simulink library "thc"  (R2021b)
settings: Solver=VariableStepAuto  StartTime=0.0  StopTime=10.0  RelTol=1e-3
undefined symbols (not defined in the file): ATHC_APTCQA_X_C, ATHC_APTCQB_X_C, ATHC_dAy_X_C, ATHC_Qeq_X_kmh, ATHC_VbaseC_X_C, ATHC_VbaseC_Y_W, ATHC_VbaseD_X_C, ATHC_VbaseH_X_C, FALSE, KTHC_ACMaxMinT_sec, KTHC_aDeice_K, KTHC_AGSDefLv_K, KTHC_AGSLv1_K, KTHC_AGSLv2_K, KTHC_AGSLv3_K, KTHC_AGSLv4_K, KTHC_AGSLv5_K, KTHC_AirIntUpdateT_sec, KTHC_APTCOneZoneMax_W, KTHC_APTCPeriod_cnt, KTHC_APTCPWMEN_flg, KTHC_APTCQMaxC_W, KTHC_APTCQminC_W, KTHC_APTCQminD_W, KTHC_APTCQminRe1_W, KTHC_APTCQminRe_W, KTHC_APTCQoffT_cnt, KTHC_APTCQonT_cnt, KTHC_APTCRiLeMaxDff_W, KTHC_APTCRiLeMinDff_W, KTHC_BatCoolT_cnt, KTHC_BatInTempDef_C, KTHC_bDeice_K, KTHC_CompMaxDeice_rpm, KTHC_CompMinDeice_rpm, KTHC_CompSotxvOp_K, KTHC_CompSotxvOpLow_rpm, KTHC_CompSpdmax_rpm, KTHC_CompSpdmaxBC1_rpm, KTHC_CompSpdmaxBC_rpm, KTHC_CompSpdmid1_rpm, KTHC_CompSpdmid2_rpm, KTHC_CompSpdmid3_rpm, KTHC_CompSpdmid_rpm, KTHC_CompSpdmin_rpm, KTHC_DAPTCQ1_W, KTHC_DAPTCQ2_W, KTHC_DAPTCQ3_W, KTHC_DcChSetTemp_C, KTHC_DehumidityEN_flg, KTHC_DeiceCycTime_K, KTHC_DriveLevelWPTCBAH1_W, KTHC_DriveLevelWPTCBAH2_W, KTHC_DriveLevelWPTCBAH3_W, KTHC_DriveLevelWPTCBAH4_W, KTHC_DriverSeatPos_flg, KTHC_DriveT1MinBAH_C, KTHC_DriveT2MaxBAH_C, KTHC_DriveT2MinBAH_C, KTHC_DriveT3MaxBAH_C ... (+379)
libraries: simulink x489
(part 14 of 17)

== system thc/THC/ThermalControl/THCM_Conctrl/CompCtrl/Enabled Subsystem ==
  sigSetTempZon1StC : Inport
  Tincar : Inport  Port=2
  Tamb : Inport  Port=3
  VINP_SmartEcoModeSW_flg : Inport  Port=4
  Enable : EnablePort
  Chart : Stateflow chart  TreatAsAtomicUnit=on
  Constant : Constant  Value=KTHC_DTymin1_K
  Constant1 : Constant  Value=KTHC_Tambmin_C
  Constant10 : Constant  Value=KTHC_T4Maxamb_C
  Constant11 : Constant  Value=KTHC_T2Minamb_C
  Constant12 : Constant  Value=KTHC_T3Minamb_C
  Constant13 : Constant  Value=KTHC_T4Minamb_C
  Constant14 : Constant  Value=KTHC_T5Minamb_C
  Constant3 : Constant  Value=KTHC_DTymin2_K
  Constant4 : Constant  Value=KTHC_DTymin3_K
  Constant5 : Constant  Value=KTHC_DTymin4_K
  Constant6 : Constant  Value=KTHC_DTymin5_K
  Constant7 : Constant  Value=KTHC_T1Maxamb_C
  Constant8 : Constant  Value=KTHC_T2Maxamb_C
  Constant9 : Constant  Value=KTHC_T3Maxamb_C
  Product : Product
  Relational Operator1 : RelationalOperator  OutDataTypeStr=boolean  RndMeth=Simplest
  Sum : Sum  Inputs=|+-
  Switch : Switch  Criteria=u2 > Threshold
  Switch1 : Switch  Criteria=u2 > Threshold
  TincarCe : Outport
  TincarCset : Outport  Port=2
  wires:
  sigSetTempZon1StC/1 -> Sum/1, TincarCset/1  "sigSetTempZon1StC"
  Tincar/1 -> Sum/2
  Switch1/1 -> Switch/1
  Switch/1 -> TincarCe/1
  Sum/1 -> Switch/3, Product/2, Switch1/3
  Constant1/1 -> Relational Operator1/2
  Relational Operator1/1 -> Switch/2
  Tamb/1 -> [Tamb]
  [Tamb] -> Chart/1(Tamb)
  Constant/1 -> Chart/2(KTHC_DTymin1_K)
  Constant3/1 -> Chart/3(KTHC_DTymin2_K)
  Constant4/1 -> Chart/4(KTHC_DTymin3_K)
  Constant5/1 -> Chart/5(KTHC_DTymin4_K)
  Constant6/1 -> Chart/6(KTHC_DTymin5_K)
  Constant7/1 -> Chart/7(KTHC_T1Maxamb_C)
  Constant8/1 -> Chart/8(KTHC_T2Maxamb_C)
  Constant9/1 -> Chart/9(KTHC_T3Maxamb_C)
  Constant10/1 -> Chart/10(KTHC_T4Maxamb_C)
  Constant11/1 -> Chart/11(KTHC_T2Minamb_C)
  Constant12/1 -> Chart/12(KTHC_T3Minamb_C)
  Constant13/1 -> Chart/13(KTHC_T4Minamb_C)
  Constant14/1 -> Chart/14(KTHC_T5Minamb_C)
  Chart/1(DTymin) -> [DTymin]
  [DTymin] -> Product/1
  [Tamb] -> Relational Operator1/1
  Product/1 -> Switch1/1
  VINP_SmartEcoModeSW_flg/1 -> Switch1/2

== system thc/THC/ThermalControl/THCM_Conctrl/CompCtrl/Enabled Subsystem1 ==
  TBMax : Inport
  Bat_In_Temp : Inport  Port=2
  Enable : EnablePort
  Chart : Stateflow chart  TreatAsAtomicUnit=on
  Constant : Constant  Value=KTHC_T1MaxBC_C
  Constant1 : Constant  Value=KTHC_T1winSetpointBC_C
  Constant10 : Constant  Value=KTHC_T3MinBC_C
  Constant11 : Constant  Value=KTHC_T3MaxBC_C
  Constant12 : Constant  Value=KTHC_T4MinBC_C
  Constant14 : Constant  Value=KTHC_T4MaxBC_C
  Constant15 : Constant  Value=KTHC_T5MinBC_C
  Constant2 : Constant  Value=KTHC_T2winSetpointBC_C
  Constant3 : Constant  Value=KTHC_T3winSetpointBC_C
  Constant4 : Constant  Value=KTHC_T4winSetpointBC_C
  Constant5 : Constant  Value=KTHC_T5winSetpointBC_C
  Constant8 : Constant  Value=KTHC_T2MinBC_C
  Constant9 : Constant  Value=KTHC_T2MaxBC_C
  Sum : Sum  Inputs=|+-
  BatIne : Outport
  BatInset : Outport  Port=2
  wires:
  TBMax/1 -> Chart/1(TBMax)
  Chart/1(Bat_In_TempSetPoint) -> BatInset/1, Sum/1  "Bat_In_TempSetPoint"
  Bat_In_Temp/1 -> Sum/2
  Sum/1 -> BatIne/1
  Constant/1 -> Chart/2(KTHC_T1MaxBC_C)
  Constant8/1 -> Chart/3(KTHC_T2MinBC_C)
  Constant9/1 -> Chart/4(KTHC_T2MaxBC_C)
  Constant10/1 -> Chart/5(KTHC_T3MinBC_C)
  Constant11/1 -> Chart/6(KTHC_T3MaxBC_C)
  Constant12/1 -> Chart/7(KTHC_T4MinBC_C)
  Constant14/1 -> Chart/8(KTHC_T4MaxBC_C)
  Constant15/1 -> Chart/9(KTHC_T5MinBC_C)
  Constant1/1 -> Chart/10(KTHC_T1winSetpointBC_C)
  Constant2/1 -> Chart/11(KTHC_T2winSetpointBC_C)
  Constant3/1 -> Chart/12(KTHC_T3winSetpointBC_C)
  Constant4/1 -> Chart/13(KTHC_T4winSetpointBC_C)
  Constant5/1 -> Chart/14(KTHC_T5winSetpointBC_C)

== system thc/THC/ThermalControl/THCM_Conctrl/CompCtrl/Enabled Subsystem2 ==
  sigSetTempZon1St : Inport
  Tincar : Inport  Port=2
  Enable : EnablePort
  Sum : Sum  Inputs=|+-
  Tincare : Outport
  Tincarset : Outport  Port=2
  wires:
  sigSetTempZon1St/1 -> Tincarset/1, Sum/1
  Sum/1 -> Tincare/1
  Tincar/1 -> Sum/2

== system thc/THC/ThermalControl/THCM_Conctrl/CompCtrl/Enabled Subsystem3 ==
  PT_Low_P2 : Inport
  PT_ Low_P2Setpoint : Inport  Port=2
  Enable : EnablePort
  Sum : Sum  Inputs=|+-
  PTLowP2e : Outport
  wires:
  PT_Low_P2/1 -> Sum/2
  PT_ Low_P2Setpoint/1 -> Sum/1
  Sum/1 -> PTLowP2e/1

== system thc/THC/ThermalControl/THCM_Conctrl/CompCtrl/Enabled Subsystem4 ==
  PT_High_P : Inport
  PT_High_PSetpoint : Inport  Port=2
  Enable : EnablePort
  Sum : Sum  Inputs=|+-
  PT_High_Pe : Outport
  wires:
  Sum/1 -> PT_High_Pe/1
  PT_High_PSetpoint/1 -> Sum/1
  PT_High_P/1 -> Sum/2

== system thc/THC/ThermalControl/THCM_Conctrl/CompCtrl/Enabled Subsystem5 ==
  PT_Low_P1 : Inport
  PT_Low_P1Setpoint : Inport  Port=2
  Enable : EnablePort
  Sum : Sum  Inputs=|+-
  PT_Low_Pe : Outport
  wires:
  PT_Low_P1/1 -> Sum/2
  PT_Low_P1Setpoint/1 -> Sum/1
  Sum/1 -> PT_Low_Pe/1

== system thc/THC/ThermalControl/THCM_Conctrl/EXV1Ctrl/EXV1PIControl ==
  x : Inport
  Reset : Inport  Port=2
  VTHC_KpEXV1SH_K : Inport  Port=3
  VTHC_KiEXV1SH_K : Inport  Port=4
  Add : Sum
  Add1 : Sum
  Constant : Constant  Value=0
  Product : Product
  Product1 : Product
  Saturation : Saturate  UpperLimit=0.1  LowerLimit=-0.9
  Switch : Switch  Criteria=u2 > Threshold
  Ts : Gain  Gain=0.1
  Unit Delay1 : UnitDelay  SampleTime=-1  HasFrameUpgradeWarning=on
  VTHC_EXV1P_K : Outport
  VTHC_EXV1I_K : Outport  Port=2
  VTHC_EXV1U_K : Outport  Port=3
  wires:
  Constant/1 -> Switch/1
  x/1 -> Product/2, Product1/1
  Product/1 -> VTHC_EXV1P_K/1, Add/1  "VTHC_EXV1P_K"
  Add/1 -> VTHC_EXV1U_K/1
  Add1/1 -> Unit Delay1/1
  Product1/1 -> Ts/1
  Switch/1 -> VTHC_EXV1I_K/1, Add/2, Add1/2  "VTHC_EXV1I_K"
  Unit Delay1/1 -> Saturation/1
  VTHC_KpEXV1SH_K/1 -> Product/1
  VTHC_KiEXV1SH_K/1 -> Product1/2
  Reset/1 -> Switch/2
  Saturation/1 -> Switch/3
  Ts/1 -> Add1/1  "VTHC_EXV1I_K"

== system thc/THC/ThermalControl/THCM_Conctrl/EXV2Ctrl/EXV2PIControl ==
  x : Inport
  Reset : Inport  Port=2
  VTHC_KpEXV2_K : Inport  Port=3
  VTHC_KiEXV2_K : Inport  Port=4
  Add : Sum
  Add1 : Sum
  Constant : Constant  Value=0
  Equal : RelationalOperator  Operator=~=  OutDataTypeStr=boolean  RndMeth=Simplest
  Product : Product
  Product1 : Product
  Saturation : Saturate  UpperLimit=0.1  LowerLimit=-0.9
  Switch : Switch  Criteria=u2 > Threshold
  Ts : Gain  Gain=0.1
  Unit Delay : UnitDelay  SampleTime=-1  HasFrameUpgradeWarning=on
  Unit Delay1 : UnitDelay  SampleTime=-1  HasFrameUpgradeWarning=on
  VTHC_EXV2P_K : Outport
  VTHC_EXV2I_K : Outport  Port=2
  VTHC_EXV2U_K : Outport  Port=3
  wires:
  Unit Delay/1 -> Equal/2
  Equal/1 -> Switch/2
  Constant/1 -> Switch/1
  x/1 -> Product1/1, Product/2
  Product/1 -> VTHC_EXV2P_K/1, Add/1  "VTHC_EXV2P_K"
  Add/1 -> VTHC_EXV2U_K/1
  Add1/1 -> Unit Delay1/1
  Product1/1 -> Ts/1
  Switch/1 -> VTHC_EXV2I_K/1, Add/2, Add1/2  "VTHC_EXV2I_K"
  Reset/1 -> Unit Delay/1, Equal/1
  VTHC_KpEXV2_K/1 -> Product/1
  VTHC_KiEXV2_K/1 -> Product1/2
  Ts/1 -> Add1/1
  Unit Delay1/1 -> Saturation/1
  Saturation/1 -> Switch/3

== system thc/THC/ThermalControl/THCM_Conctrl/Subsystem1/SensorErrorHandle1 ==
  DataIn : Inport
  SensorError : Inport  Port=2
  PresetValue : Inport  Port=3
  Constant : Constant  Value=KTHC_ErrHandleEN_flg
  Logical Operator : Logic  AllPortsSameDT=off  OutDataTypeStr=boolean
  Switch : Switch  Criteria=u2 > Threshold
  DataOut : Outport
  wires:
  PresetValue/1 -> Switch/1
  DataIn/1 -> Switch/3
  Switch/1 -> DataOut/1
  Logical Operator/1 -> Switch/2
  SensorError/1 -> Logical Operator/1
  Constant/1 -> Logical Operator/2

== system thc/THC/ThermalControl/THCM_Conctrl/Subsystem1/SensorErrorHandle2 ==
  DataIn : Inport
  SensorError : Inport  Port=2
  PresetValue : Inport  Port=3
  Constant : Constant  Value=KTHC_ErrHandleEN_flg
  Logical Operator : Logic  AllPortsSameDT=off  OutDataTypeStr=boolean
  Switch : Switch  Criteria=u2 > Threshold
  DataOut : Outport
  wires:
  Constant/1 -> Logical Operator/2
  SensorError/1 -> Logical Operator/1
  Logical Operator/1 -> Switch/2
  Switch/1 -> DataOut/1
  DataIn/1 -> Switch/3
  PresetValue/1 -> Switch/1

== system thc/THC/ThermalControl/THCM_Conctrl/Subsystem1/SensorErrorHandle3 ==
  DataIn : Inport
  SensorError : Inport  Port=2
  PresetValue : Inport  Port=3
  Constant : Constant  Value=KTHC_ErrHandleEN_flg
  Logical Operator : Logic  AllPortsSameDT=off  OutDataTypeStr=boolean
  Switch : Switch  Criteria=u2 > Threshold
  DataOut : Outport
  wires:
  PresetValue/1 -> Switch/1
  DataIn/1 -> Switch/3
  Switch/1 -> DataOut/1
  Logical Operator/1 -> Switch/2
  SensorError/1 -> Logical Operator/1
  Constant/1 -> Logical Operator/2

== system thc/THC/ThermalControl/THCM_Conctrl/Subsystem1/SensorErrorHandle4 ==
  DataIn : Inport
  SensorError : Inport  Port=2
  PresetValue : Inport  Port=3
  Constant : Constant  Value=KTHC_ErrHandleEN_flg
  Logical Operator : Logic  AllPortsSameDT=off  OutDataTypeStr=boolean
  Switch : Switch  Criteria=u2 > Threshold
  DataOut : Outport
  wires:
  Constant/1 -> Logical Operator/2
  SensorError/1 -> Logical Operator/1
  Logical Operator/1 -> Switch/2
  Switch/1 -> DataOut/1
  DataIn/1 -> Switch/3
  PresetValue/1 -> Switch/1

== system thc/THC/ThermalControl/THCM_Conctrl/Subsystem1/SensorErrorHandle5 ==
  DataIn : Inport
  SensorError : Inport  Port=2
  PresetValue : Inport  Port=3
  Constant : Constant  Value=KTHC_ErrHandleEN_flg
  Logical Operator : Logic  AllPortsSameDT=off  OutDataTypeStr=boolean
  Switch : Switch  Criteria=u2 > Threshold
  DataOut : Outport
  wires:
  PresetValue/1 -> Switch/1
  DataIn/1 -> Switch/3
  Switch/1 -> DataOut/1
  Logical Operator/1 -> Switch/2
  SensorError/1 -> Logical Operator/1
  Constant/1 -> Logical Operator/2

== system thc/THC/ThermalControl/THCM_Conctrl/Subsystem1/SensorErrorHandle9 ==
  DataIn : Inport
  SensorError : Inport  Port=2
  PresetValue : Inport  Port=3
  Constant : Constant  Value=KTHC_ErrHandleEN_flg
  Logical Operator : Logic  AllPortsSameDT=off  OutDataTypeStr=boolean
  Switch : Switch  Criteria=u2 > Threshold
  DataOut : Outport
  wires:
  Constant/1 -> Logical Operator/2
  SensorError/1 -> Logical Operator/1
  Logical Operator/1 -> Switch/2
  Switch/1 -> DataOut/1
  DataIn/1 -> Switch/3
  PresetValue/1 -> Switch/1

== system thc/THC/ThermalControl/THCM_Conctrl/Subsystem2/SensorErrorHandle9 ==
  DataIn : Inport
  SensorError : Inport  Port=2
  PresetValue : Inport  Port=3
  Constant : Constant  Value=KTHC_ErrHandleEN_flg
  Logical Operator : Logic  AllPortsSameDT=off  OutDataTypeStr=boolean
  Switch : Switch  Criteria=u2 > Threshold
  DataOut : Outport
  wires:
  Constant/1 -> Logical Operator/2
  SensorError/1 -> Logical Operator/1
  Logical Operator/1 -> Switch/2
  Switch/1 -> DataOut/1
  DataIn/1 -> Switch/3
  PresetValue/1 -> Switch/1

== system thc/THC/ThermalControl/THCM_Conctrl/Subsystem3/Subsystem1 ==
  "VINP_EWPBlockError_enum " : Inport
  VINP_EWPOverCurrError_enum : Inport  Port=2
  Add{,1..3} (4 alike) : Sum
  Constant{,1,6,10..11} (5 alike) : Constant  Value=0
  Constant12 : Constant  Value=KTHC_EWPRetryWarnT_cnt
  Constant13 : Constant  Value=KTHC_EWPErrHandleEN_flg
  Constant14 : Constant  Value=KTHC_EWPTotalRetryT_cnt
  Constant2 : Constant  Value=KTHC_EWPErrorT_cnt
  Constant3 : Constant
  Constant4 : Constant  Value=KTHC_EWPpauseT_cnt
  Constant5 : Constant  Value=KTHC_EWPretryT_cnt
  Constant7 : Constant
  Constant8 : Constant  Value=KTHC_EWPpauseT_cnt
  Constant9 : Constant
  Data Type Conversion{,1..9} (10 alike) : DataTypeConversion  OutDataTypeStr=uint16
  Data Type Conversion10 : DataTypeConversion  OutDataTypeStr=boolean
  Detect Increase : simulink/Logic and Bit Operations/Detect Increase  vinit=0.0  OutDataTypeStr=boolean
  Logical Operator : Logic  Operator=OR  AllPortsSameDT=off  OutDataTypeStr=boolean
  Logical Operator1 : Logic  Operator=NOT  AllPortsSameDT=off  OutDataTypeStr=boolean
  Logical Operator2 : Logic  Operator=OR  AllPortsSameDT=off  OutDataTypeStr=boolean
  Logical Operator3 : Logic  AllPortsSameDT=off  OutDataTypeStr=boolean
  Logical Operator4 : Logic  AllPortsSameDT=off  OutDataTypeStr=boolean
  Logical Operator5 : Logic  Operator=OR  AllPortsSameDT=off  OutDataTypeStr=boolean
  Relational Operator : RelationalOperator  OutDataTypeStr=boolean  RndMeth=Simplest
  Relational Operator1 : RelationalOperator  OutDataTypeStr=boolean  RndMeth=Simplest
  Relational Operator2 : RelationalOperator  Operator=<  OutDataTypeStr=boolean  RndMeth=Simplest
  Relational Operator3 : RelationalOperator  Operator=>  OutDataTypeStr=boolean  RndMeth=Simplest
  Relational Operator4 : RelationalOperator  Operator=>  OutDataTypeStr=boolean  RndMeth=Simplest
  Saturation : Saturate  UpperLimit=1000  LowerLimit=0
  Switch{,1..4} (5 alike) : Switch  Criteria=u2 > Threshold
  Unit Delay : UnitDelay  SampleTime=-1  HasFrameUpgradeWarning=on
  Unit Delay1 : UnitDelay  SampleTime=-1  HasFrameUpgradeWarning=on
  Unit Delay2 : UnitDelay  SampleTime=-1  HasFrameUpgradeWarning=on
  EWPerror : Outport
  EWPpause : Outport  Port=2
  EWPBUflag : Outport  Port=3
  wires:
  "VINP_EWPBlockError_enum "/1 -> Logical Operator/1
  VINP_EWPOverCurrError_enum/1 -> Logical Operator/2
  Logical Operator/1 -> Logical Operator4/2
  Unit Delay/1 -> Relational Operator/1, Add/1
  Add/1 -> Switch/1
  Constant/1 -> Data Type Conversion/1
  Switch/1 -> Data Type Conversion2/1
  Data Type Conversion1/1 -> Switch/3
  Constant1/1 -> Data Type Conversion1/1
  Data Type Conversion2/1 -> Unit Delay/1
  Switch1/1 -> Add/2
  Data Type Conversion/1 -> Switch1/1
  Constant2/1 -> Relational Operator/2
  Relational Operator/1 -> [EWPerror], EWPerror/1, Switch1/2
  Constant3/1 -> Data Type Conversion3/1
  Data Type Conversion3/1 -> Switch1/3
  Constant4/1 -> Add1/1
  Constant5/1 -> Add1/2
  Add1/1 -> [Period]
  Constant7/1 -> Data Type Conversion5/1
  Data Type Conversion5/1 -> Add2/2
  Unit Delay2/1 -> Add2/1
  Switch3/1 -> Relational Operator2/1, Unit Delay2/1
  Relational Operator1/1 -> Logical Operator2/1
  [Period] -> Relational Operator1/2
  Add2/1 -> Switch3/3, Relational Operator1/1
  Data Type Conversion4/1 -> Switch3/1
  Constant6/1 -> Data Type Conversion4/1
  [EWPerror] -> Logical Operator1/1
  Logical Operator2/1 -> Switch3/2
  Logical Operator1/1 -> Logical Operator2/2
  Constant8/1 -> Relational Operator2/2
  Relational Operator2/1 -> Logical Operator3/1
  [EWPerror] -> Logical Operator3/2
  Logical Operator3/1 -> Logical Operator5/1, Detect Increase/1
  Detect Increase/1 -> Switch2/2
  Constant9/1 -> Data Type Conversion6/1
  Data Type Conversion6/1 -> Switch2/1
  Data Type Conversion7/1 -> Switch2/3
  Constant10/1 -> Data Type Conversion7/1
  Switch2/1 -> Add3/1
  Unit Delay1/1 -> Add3/2
  Switch4/1 -> Data Type Conversion8/1
  Data Type Conversion8/1 -> Saturation/1
  Saturation/1 -> Relational Operator4/1, Unit Delay1/1, Relational Operator3/1
  Add3/1 -> Switch4/1
  [EWPerror] -> Switch4/2
  Constant11/1 -> Data Type Conversion9/1
  Data Type Conversion9/1 -> Switch4/3
  Constant12/1 -> Relational Operator3/2
  Relational Operator3/1 -> EWPBUflag/1
  Logical Operator4/1 -> Switch/2
  Constant13/1 -> Data Type Conversion10/1
  Data Type Conversion10/1 -> Logical Operator4/1
  Relational Operator4/1 -> [StopRetry]
  Logical Operator5/1 -> EWPpause/1
  [StopRetry] -> Logical Operator5/2
  Constant14/1 -> Relational Operator4/2

== system thc/THC/ThermalControl/THCM_Conctrl/Subsystem3/Subsystem2 ==
  "VINP_EWPBlockError_enum " : Inport
  VINP_EWPOverCurrError_enum : Inport  Port=2
  Add{,1..3} (4 alike) : Sum
  Constant{,1,6,10..11} (5 alike) : Constant  Value=0
  Constant12 : Constant  Value=KTHC_EWPRetryWarnT_cnt
  Constant13 : Constant  Value=KTHC_EWPErrHandleEN_flg
  Constant14 : Constant  Value=KTHC_EWPTotalRetryT_cnt
  Constant2 : Constant  Value=KTHC_EWPErrorT_cnt
  Constant3 : Constant
  Constant4 : Constant  Value=KTHC_EWPpauseT_cnt
  Constant5 : Constant  Value=KTHC_EWPretryT_cnt
  Constant7 : Constant
  Constant8 : Constant  Value=KTHC_EWPpauseT_cnt
  Constant9 : Constant
  Data Type Conversion{,1..9} (10 alike) : DataTypeConversion  OutDataTypeStr=uint16
  Data Type Conversion10 : DataTypeConversion  OutDataTypeStr=boolean
  Detect Increase : simulink/Logic and Bit Operations/Detect Increase  vinit=0.0  OutDataTypeStr=boolean
  Logical Operator : Logic  Operator=OR  AllPortsSameDT=off  OutDataTypeStr=boolean
  Logical Operator1 : Logic  Operator=NOT  AllPortsSameDT=off  OutDataTypeStr=boolean
  Logical Operator2 : Logic  Operator=OR  AllPortsSameDT=off  OutDataTypeStr=boolean
  Logical Operator3 : Logic  AllPortsSameDT=off  OutDataTypeStr=boolean
  Logical Operator4 : Logic  AllPortsSameDT=off  OutDataTypeStr=boolean
  Logical Operator5 : Logic  Operator=OR  AllPortsSameDT=off  OutDataTypeStr=boolean
  Relational Operator : RelationalOperator  OutDataTypeStr=boolean  RndMeth=Simplest
  Relational Operator1 : RelationalOperator  OutDataTypeStr=boolean  RndMeth=Simplest
  Relational Operator2 : RelationalOperator  Operator=<  OutDataTypeStr=boolean  RndMeth=Simplest
  Relational Operator3 : RelationalOperator  Operator=>  OutDataTypeStr=boolean  RndMeth=Simplest
  Relational Operator4 : RelationalOperator  Operator=>  OutDataTypeStr=boolean  RndMeth=Simplest
  Saturation : Saturate  UpperLimit=1000  LowerLimit=0
  Switch{,1..4} (5 alike) : Switch  Criteria=u2 > Threshold
  Unit Delay : UnitDelay  SampleTime=-1  HasFrameUpgradeWarning=on
  Unit Delay1 : UnitDelay  SampleTime=-1  HasFrameUpgradeWarning=on
  Unit Delay2 : UnitDelay  SampleTime=-1  HasFrameUpgradeWarning=on
  EWPerror : Outport
  EWPpause : Outport  Port=2
  EWPBUflag : Outport  Port=3
  wires:
  Constant14/1 -> Relational Operator4/2
  [StopRetry] -> Logical Operator5/2
  Logical Operator5/1 -> EWPpause/1
  Relational Operator4/1 -> [StopRetry]
  Data Type Conversion10/1 -> Logical Operator4/1
  Constant13/1 -> Data Type Conversion10/1
  Logical Operator4/1 -> Switch/2
  Relational Operator3/1 -> EWPBUflag/1
  Constant12/1 -> Relational Operator3/2
  Data Type Conversion9/1 -> Switch4/3
  Constant11/1 -> Data Type Conversion9/1
  [EWPerror] -> Switch4/2
  Add3/1 -> Switch4/1
  Saturation/1 -> Relational Operator3/1, Unit Delay1/1, Relational Operator4/1
  Data Type Conversion8/1 -> Saturation/1
  Switch4/1 -> Data Type Conversion8/1
  Unit Delay1/1 -> Add3/2
  Switch2/1 -> Add3/1
  Constant10/1 -> Data Type Conversion7/1
  Data Type Conversion7/1 -> Switch2/3
  Data Type Conversion6/1 -> Switch2/1
  Constant9/1 -> Data Type Conversion6/1
  Detect Increase/1 -> Switch2/2
  Logical Operator3/1 -> Detect Increase/1, Logical Operator5/1
  [EWPerror] -> Logical Operator3/2
  Relational Operator2/1 -> Logical Operator3/1
  Constant8/1 -> Relational Operator2/2
  Logical Operator1/1 -> Logical Operator2/2
  Logical Operator2/1 -> Switch3/2
  [EWPerror] -> Logical Operator1/1
  Constant6/1 -> Data Type Conversion4/1
  Data Type Conversion4/1 -> Switch3/1
  Add2/1 -> Relational Operator1/1, Switch3/3
  [Period] -> Relational Operator1/2
  Relational Operator1/1 -> Logical Operator2/1
  Switch3/1 -> Unit Delay2/1, Relational Operator2/1
  Unit Delay2/1 -> Add2/1
  Data Type Conversion5/1 -> Add2/2
  Constant7/1 -> Data Type Conversion5/1
  Add1/1 -> [Period]
  Constant5/1 -> Add1/2
  Constant4/1 -> Add1/1
  Data Type Conversion3/1 -> Switch1/3
  Constant3/1 -> Data Type Conversion3/1
  Relational Operator/1 -> Switch1/2, EWPerror/1, [EWPerror]
  Constant2/1 -> Relational Operator/2
  Data Type Conversion/1 -> Switch1/1
  Switch1/1 -> Add/2
  Data Type Conversion2/1 -> Unit Delay/1
  Constant1/1 -> Data Type Conversion1/1
  Data Type Conversion1/1 -> Switch/3
  Switch/1 -> Data Type Conversion2/1
  Constant/1 -> Data Type Conversion/1
  Add/1 -> Switch/1
  Unit Delay/1 -> Add/1, Relational Operator/1
  Logical Operator/1 -> Logical Operator4/2
  VINP_EWPOverCurrError_enum/1 -> Logical Operator/2
  "VINP_EWPBlockError_enum "/1 -> Logical Operator/1

== system thc/THC/ThermalControl/THCM_Conctrl/Subsystem3/Subsystem3 ==
  "VINP_EWPBlockError_enum " : Inport
  VINP_EWPOverCurrError_enum : Inport  Port=2
  Add{,1..3} (4 alike) : Sum
  Constant{,1,6,10..11} (5 alike) : Constant  Value=0
  Constant12 : Constant  Value=KTHC_EWPRetryWarnT_cnt
  Constant13 : Constant  Value=KTHC_EWPErrHandleEN_flg
  Constant14 : Constant  Value=KTHC_EWPTotalRetryT_cnt
  Constant2 : Constant  Value=KTHC_EWPErrorT_cnt
  Constant3 : Constant
  Constant4 : Constant  Value=KTHC_EWPpauseT_cnt
  Constant5 : Constant  Value=KTHC_EWPretryT_cnt
  Constant7 : Constant
  Constant8 : Constant  Value=KTHC_EWPpauseT_cnt
  Constant9 : Constant
  Data Type Conversion{,1..9} (10 alike) : DataTypeConversion  OutDataTypeStr=uint16
  Data Type Conversion10 : DataTypeConversion  OutDataTypeStr=boolean
  Detect Increase : simulink/Logic and Bit Operations/Detect Increase  vinit=0.0  OutDataTypeStr=boolean
  Logical Operator : Logic  Operator=OR  AllPortsSameDT=off  OutDataTypeStr=boolean
  Logical Operator1 : Logic  Operator=NOT  AllPortsSameDT=off  OutDataTypeStr=boolean
  Logical Operator2 : Logic  Operator=OR  AllPortsSameDT=off  OutDataTypeStr=boolean
  Logical Operator3 : Logic  AllPortsSameDT=off  OutDataTypeStr=boolean
  Logical Operator4 : Logic  AllPortsSameDT=off  OutDataTypeStr=boolean
  Logical Operator5 : Logic  Operator=OR  AllPortsSameDT=off  OutDataTypeStr=boolean
  Relational Operator : RelationalOperator  OutDataTypeStr=boolean  RndMeth=Simplest
  Relational Operator1 : RelationalOperator  OutDataTypeStr=boolean  RndMeth=Simplest
  Relational Operator2 : RelationalOperator  Operator=<  OutDataTypeStr=boolean  RndMeth=Simplest
  Relational Operator3 : RelationalOperator  Operator=>  OutDataTypeStr=boolean  RndMeth=Simplest
  Relational Operator4 : RelationalOperator  Operator=>  OutDataTypeStr=boolean  RndMeth=Simplest
  Saturation : Saturate  UpperLimit=1000  LowerLimit=0
  Switch{,1..4} (5 alike) : Switch  Criteria=u2 > Threshold
  Unit Delay : UnitDelay  SampleTime=-1  HasFrameUpgradeWarning=on
  Unit Delay1 : UnitDelay  SampleTime=-1  HasFrameUpgradeWarning=on
  Unit Delay2 : UnitDelay  SampleTime=-1  HasFrameUpgradeWarning=on
  EWPerror : Outport
  EWPpause : Outport  Port=2
  EWPBUflag : Outport  Port=3
  wires:
  Constant14/1 -> Relational Operator4/2
  [StopRetry] -> Logical Operator5/2
  Logical Operator5/1 -> EWPpause/1
  Relational Operator4/1 -> [StopRetry]
  Data Type Conversion10/1 -> Logical Operator4/1
  Constant13/1 -> Data Type Conversion10/1
  Logical Operator4/1 -> Switch/2
  Relational Operator3/1 -> EWPBUflag/1
  Constant12/1 -> Relational Operator3/2
  Data Type Conversion9/1 -> Switch4/3
  Constant11/1 -> Data Type Conversion9/1
  [EWPerror] -> Switch4/2
  Add3/1 -> Switch4/1
  Saturation/1 -> Relational Operator3/1, Unit Delay1/1, Relational Operator4/1
  Data Type Conversion8/1 -> Saturation/1
  Switch4/1 -> Data Type Conversion8/1
  Unit Delay1/1 -> Add3/2
  Switch2/1 -> Add3/1
  Constant10/1 -> Data Type Conversion7/1
  Data Type Conversion7/1 -> Switch2/3
  Data Type Conversion6/1 -> Switch2/1
  Constant9/1 -> Data Type Conversion6/1
  Detect Increase/1 -> Switch2/2
  Logical Operator3/1 -> Detect Increase/1, Logical Operator5/1
  [EWPerror] -> Logical Operator3/2
  Relational Operator2/1 -> Logical Operator3/1
  Constant8/1 -> Relational Operator2/2
  Logical Operator1/1 -> Logical Operator2/2
  Logical Operator2/1 -> Switch3/2
  [EWPerror] -> Logical Operator1/1
  Constant6/1 -> Data Type Conversion4/1
  Data Type Conversion4/1 -> Switch3/1
  Add2/1 -> Relational Operator1/1, Switch3/3
  [Period] -> Relational Operator1/2
  Relational Operator1/1 -> Logical Operator2/1
  Switch3/1 -> Unit Delay2/1, Relational Operator2/1
  Unit Delay2/1 -> Add2/1
  Data Type Conversion5/1 -> Add2/2
  Constant7/1 -> Data Type Conversion5/1
  Add1/1 -> [Period]
  Constant5/1 -> Add1/2
  Constant4/1 -> Add1/1
  Data Type Conversion3/1 -> Switch1/3
  Constant3/1 -> Data Type Conversion3/1
  Relational Operator/1 -> Switch1/2, EWPerror/1, [EWPerror]
  Constant2/1 -> Relational Operator/2
  Data Type Conversion/1 -> Switch1/1
  Switch1/1 -> Add/2
  Data Type Conversion2/1 -> Unit Delay/1
  Constant1/1 -> Data Type Conversion1/1
  Data Type Conversion1/1 -> Switch/3
  Switch/1 -> Data Type Conversion2/1
  Constant/1 -> Data Type Conversion/1
  Add/1 -> Switch/1
  Unit Delay/1 -> Add/1, Relational Operator/1
  Logical Operator/1 -> Logical Operator4/2
  VINP_EWPOverCurrError_enum/1 -> Logical Operator/2
  "VINP_EWPBlockError_enum "/1 -> Logical Operator/1

== stateflow chart thc/THC/ThermalControl/THCM_Conctrl/APTC/APTCPWMControl/Chart ==
  state APTC
    en:
    Wout=Win;
    du:
    Wout=Win;
  state APTCPWM
    (default) -> (junction 5) : {Tcnt=0;OnT=0;OffT=0;}
    APTCPWM -> (junction 5) [order 1]
    (junction 5) -> (junction 7) [order 1] : [Win==0]{Wout=0;}
    (junction 5) -> (junction 9) [order 2]
    (junction 7) -> (junction 11)
    (junction 9) -> (junction 11) [order 1] : [Win>Wmin]{Wout=Win;}
    (junction 9) -> (junction 54) [order 2]
    (junction 11) -> (junction 56)
    (junction 54) -> (junction 56) [order 1] : [Wout>Wmin]{Tcnt=0;Wout=0;....
        | OnT=Tp*Win/Wmin;OffT=Tp-OnT;}
    (junction 54) -> (junction 13) [order 2]
    (junction 56) -> (junction 15)
    (junction 13) -> (junction 15) [order 1] : [Wout>0&&Tcnt>=OnT]
        | {Tcnt=0;Wout=0;}
    (junction 13) -> (junction 17) [order 2]
    (junction 15) -> (junction 19)
    (junction 17) -> (junction 19) [order 1] : [Wout==0&&Tcnt>=OffT]
        | {Tcnt=0;Wout=Wmin;....
        | OnT=Tp*Win/Wmin;OffT=Tp-OnT;}
    (junction 17) -> (junction 26) [order 2]
    (junction 19) -> (junction 28)
    (junction 26) -> (junction 28)
    (junction 28) -> (junction 31) [order 2] : {Tcnt=Tcnt+1;}
    (junction 28) -> (junction 33) [order 1] : [Tcnt>Tp||(OnT==0&&OffT==0)]
        | {Tcnt=0;OnT=0;OffT=0;}
  (default) -> (junction 50)
  (junction 50) -> APTC [order 1] : [!KTHC_APTCPWMEN_flg]
  (junction 50) -> APTCPWM [order 2]
  APTCPWM -> APTC [order 1] : [!KTHC_APTCPWMEN_flg]
  APTC -> APTCPWM : [KTHC_APTCPWMEN_flg]
  data: OnT local uint16; OffT local uint16; Tcnt local uint16; Win input; Wout output uint16; Tp input uint16; Wmin input; KTHC_APTCPWMEN_flg input

== stateflow chart thc/THC/ThermalControl/THCM_Conctrl/Chart2 ==
  state FactorSolar1
    en:FactorSolar=0.88;Blowersolar=1000;
    state Low
    state Mid
    (default) -> FactorSolar1.Mid
    FactorSolar1.Mid -> FactorSolar1.Low : [Solar<950]
    FactorSolar1.Low -> FactorSolar1.Mid [order 1] : [Solar>=950]
  state FactorSolar2
    en:FactorSolar=0.90;Blowersolar=860;
    state Low
    state Mid
    state High
    (default) -> FactorSolar2.Mid
    FactorSolar2.Mid -> FactorSolar2.High [order 2] : [Solar>1000]
    FactorSolar2.Mid -> FactorSolar2.Low [order 1] : [Solar<800]
    FactorSolar2.Low -> FactorSolar2.Mid [order 1] : [Solar>=800]
    FactorSolar2.High -> FactorSolar2.Mid [order 2] : [Solar<=1000]
  state FactorSolar3
    en:FactorSolar=0.92;Blowersolar=715;
    state Low
    state Mid
    state High
    (default) -> FactorSolar3.Mid
    FactorSolar3.Mid -> FactorSolar3.High [order 2] : [Solar>850]
    FactorSolar3.Mid -> FactorSolar3.Low [order 1] : [Solar<650]
    FactorSolar3.Low -> FactorSolar3.Mid [order 1] : [Solar>=650]
    FactorSolar3.High -> FactorSolar3.Mid [order 1] : [Solar<=850]
  state FactorSolar4
    en:FactorSolar=0.94;Blowersolar=570;
    state Low
    state Mid
    state High
    (default) -> FactorSolar4.Mid
    FactorSolar4.Mid -> FactorSolar4.High [order 2] : [Solar>700]
    FactorSolar4.Mid -> FactorSolar4.Low [order 1] : [Solar<500]
    FactorSolar4.Low -> FactorSolar4.Mid [order 1] : [Solar>=500]
    FactorSolar4.High -> FactorSolar4.Mid [order 1] : [Solar<=700]
  state FactorSolar5
    en:FactorSolar=0.96;Blowersolar=430;
    state Low
    state Mid
    state High
    (default) -> FactorSolar5.Mid
    FactorSolar5.Mid -> FactorSolar5.High [order 2] : [Solar>550]
    FactorSolar5.Mid -> FactorSolar5.Low [order 1] : [Solar<350]
    FactorSolar5.Low -> FactorSolar5.Mid [order 1] : [Solar>=350]
    FactorSolar5.High -> FactorSolar5.Mid [order 1] : [Solar<=550]
  state FactorSolar6
    en:FactorSolar=0.98;Blowersolar=285;
    state Low
    state Mid
    state High
    (default) -> FactorSolar6.Mid
    FactorSolar6.Mid -> FactorSolar6.High [order 2] : [Solar>400]
    FactorSolar6.Mid -> FactorSolar6.Low [order 1] : [Solar<200]
    FactorSolar6.Low -> FactorSolar6.Mid : [Solar>=200]
    FactorSolar6.High -> FactorSolar6.Mid [order 1] : [Solar<=400]
  state FactorSolar7
    en:FactorSolar=1;Blowersolar=100;
    state Mid
    state High
    (default) -> FactorSolar7.Mid
    FactorSolar7.Mid -> FactorSolar7.High : [Solar>250]
    FactorSolar7.High -> FactorSolar7.Mid [order 1] : [Solar<=250]
  (default) -> (junction 9)
  (junction 9) -> FactorSolar1 [order 1] : [Solar>950]
  (junction 9) -> (junction 11) [order 2]
  FactorSolar1.Low -> FactorSolar2 [order 2] : [after(KTHC_SolarDebounceT_sec*10,tick)]
  FactorSolar2.High -> FactorSolar1 [order 1] : [after(KTHC_SolarDebounceT_sec*10,tick)]
  (junction 11) -> FactorSolar2 [order 1] : [Solar>800]
  (junction 11) -> (junction 14) [order 2]
  FactorSolar2.Low -> FactorSolar3 [order 2] : [after(KTHC_SolarDebounceT_sec*10,tick)]
  FactorSolar3.High -> FactorSolar2 [order 2] : [after(KTHC_SolarDebounceT_sec*10,tick)]
  (junction 14) -> FactorSolar3 [order 1] : [Solar>650]
  (junction 14) -> (junction 17) [order 2]
  FactorSolar3.Low -> FactorSolar4.Low [order 2] : [after(KTHC_SolarDebounceT_sec*10,tick)]
  FactorSolar4.High -> FactorSolar3 [order 2] : [after(KTHC_SolarDebounceT_sec*10,tick)]
  (junction 17) -> FactorSolar4 [order 1] : [Solar>500]
  (junction 17) -> (junction 20) [order 2]
  FactorSolar4.Low -> FactorSolar5.Low [order 2] : [after(KTHC_SolarDebounceT_sec*10,tick)]
  FactorSolar5.High -> FactorSolar4 [order 2] : [after(KTHC_SolarDebounceT_sec*10,tick)]
  (junction 20) -> FactorSolar5 [order 1] : [Solar>350]
  (junction 20) -> (junction 23) [order 2]
  FactorSolar5.Low -> FactorSolar6.Low [order 2] : [after(KTHC_SolarDebounceT_sec*10,tick)]
  FactorSolar6.High -> FactorSolar5 [order 2] : [after(KTHC_SolarDebounceT_sec*10,tick)]
  (junction 23) -> FactorSolar6 [order 1] : [Solar>200]
  (junction 23) -> (junction 26) [order 2]
  FactorSolar7.High -> FactorSolar6 [order 2] : [after(KTHC_SolarDebounceT_sec*10,tick)]
  (junction 26) -> FactorSolar7
  data: Solar input; FactorSolar output single; KTHC_SolarDebounceT_sec input; Blowersolar output

== stateflow chart thc/THC/ThermalControl/THCM_Conctrl/BlowerCtrl/SlowIncrease ==
  state OFF
    en:Bout=0;
  state ON
    state Increase
      en:Bout=KTHC_VBstep_K;
      du:Bout=Bout+KTHC_VBstep_K;
    state Operating
      en:Bout=Bin;
      du:Bout=Bin;
    Increase -> Operating : [Bin<Bout+KTHC_VBstep_K]
  (default) -> OFF
  OFF -> Increase : [Bin>0]
  ON -> OFF : [Bin<=0]
  data: Bin input; Bout output; KTHC_VBstep_K input

== stateflow chart thc/THC/ThermalControl/THCM_Conctrl/Chart ==
  state CabinModeDet [parallel]
    settings: executionOrder=1
    state CabinMode4or5
    state Heating
    state Else
    (default) -> (junction 50)
    (junction 50) -> CabinMode4or5 [order 1] : [CabinMode==4||CabinMode==5]
    (junction 50) -> (junction 54) [order 2]
    CabinMode4or5 -> Heating [order 1] : [CabinMode==8||CabinMode==9]
        | {Balance=true;}
    (junction 65) -> CabinMode4or5 : [CabinMode==4||....
        | CabinMode==5]
    CabinMode4or5 -> Else [order 2] : [CabinMode!=4&&....
        | CabinMode!=5]
    Heating -> (junction 65) [order 1]
    (junction 54) -> Heating [order 1] : [CabinMode==8||CabinMode==9]
    (junction 54) -> Else [order 2]
    Else -> (junction 65) [order 2]
    Else -> Heating [order 1] : [CabinMode==8||CabinMode==9]
    Heating -> Else [order 2] : [CabinMode!=8&&....
        | CabinMode!=9]
  state HighPBalance [parallel]
    settings: executionOrder=2
    state DeCrease
      en:CompOut=CompOut-Step;
      du:CompOut=CompOut-Step;
    state Finish
      en:CompOut=CompIn;
      SOTXVout=SOTXV;
      du:CompOut=CompIn;
      SOTXVout=SOTXV;
    (default) -> (junction 9)
    HighPBalance -> (junction 9) : [Balance]{Balance=false;}
    (junction 9) -> DeCrease [order 1] : [CompOut>KTHC_CompSotxvOpLow_rpm&&....
        | PT_High_P>KTHC_SotxvProHi_kPa]....
        | {Step=(CompOut-KTHC_CompSotxvOpLow_rpm)/KTHC_CompSotxvOp_K;}
    (junction 9) -> (junction 14) [order 2]
    DeCrease -> Finish : [CompOut<KTHC_CompSotxvOpLow_rpm&&....
        | PT_High_P<KTHC_SotxvProLo_kPa]
    (junction 14) -> Finish
  data: CabinMode input; CompIn input; Step local double; CompOut output =0; SOTXVout output boolean =false; KTHC_CompSotxvOpLow_rpm input; KTHC_CompSotxvOp_K input; KTHC_SotxvProHi_kPa input; KTHC_SotxvProLo_kPa input; PT_High_P input; Balance local boolean; SOTXV input

== stateflow chart thc/THC/ThermalControl/THCM_Conctrl/BlowerCtrl/Enabled Subsystem1/Chart2 ==
  state Voffset [parallel]
    settings: executionOrder=2
    state ACOFF
      state POWERon
        en:Voffset=Vmanual;
        du:Voffset=Vmanual;
      state OFF
        en:Voffset=0;
      (default) -> (junction 8)
      (junction 8) -> POWERon [order 2]
      (junction 8) -> OFF [order 1] : [CabinMode==0||....
          | PwrSta<=3]
      OFF -> POWERon : [CabinMode~=0&&PwrSta>3]
      POWERon -> OFF : [CabinMode==0||....
          | PwrSta<=3]
    state ACON
      state Defrst
        state Manual
          en:Voffset=Vmanual;
          du:Voffset=Vmanual;
        state Auto
          en:Voffset=KTHC_VBlowerdfog_K;
        (default) -> (junction 56)
        (junction 56) -> Voffset.ACON.Defrst.Auto [order 1] : [ACAuto]
        (junction 56) -> Voffset.ACON.Defrst.Manual [order 2]
        Voffset.ACON.Defrst.Manual -> Voffset.ACON.Defrst.Auto : [ACAuto]
        Voffset.ACON.Defrst.Auto -> Voffset.ACON.Defrst.Manual : [!ACAuto]
      state DefrstOFF
        state Auto
          state DontCorrect3
            en:Voffset=KTHC_VBlowerSetLow_K;
          state Vbase1
            en:Voffset=KTHC_VBlowerDcCh_K;
          state Vbase
            en:Voffset=Vbase;
            du:Voffset=Vbase;
          (default) -> (junction 105)
          (junction 105) -> DontCorrect3 [order 1] : [CabinMode==3&&....
              | (ACSubMode==6||ACSubMode==7||ACSubMode==0)]
          Voffset.ACON.DefrstOFF.Auto -> (junction 105) [order 1] : [hasChanged(CabinMode)||....
              | hasChanged(ACSubMode)]
          (junction 105) -> (junction 304) [order 2]
          (junction 304) -> Vbase1 [order 1] : [CabinMode==11]
          (junction 304) -> (junction 293) [order 2]
          (junction 293) -> Voffset.ACON.DefrstOFF.Auto.Vbase
        state Manual
          state DontCorrect
            en:Voffset=Vmanual;
            du:Voffset=Vmanual;
          state Vbase
            en:Voffset=Vbase;
            du:Voffset=Vbase;
          (default) -> (junction 83)
          Voffset.ACON.DefrstOFF.Manual -> (junction 83) [order 1] : [hasChanged(CabinMode)||....
              | hasChanged(ACSubMode)]
          (junction 83) -> DontCorrect [order 1] : [(CabinMode==3&&ACSubMode>=4)||CabinMode==7]
          (junction 83) -> (junction 91) [order 2]
          (junction 91) -> Voffset.ACON.DefrstOFF.Manual.Vbase
        (default) -> (junction 76)
        (junction 76) -> Voffset.ACON.DefrstOFF.Manual [order 2]
        (junction 76) -> Voffset.ACON.DefrstOFF.Auto [order 1] : [ACAuto]
        Voffset.ACON.DefrstOFF.Manual -> Voffset.ACON.DefrstOFF.Auto [order 1] : [ACAuto]
        Voffset.ACON.DefrstOFF.Auto -> Voffset.ACON.DefrstOFF.Manual [order 1] : [!ACAuto]
      (default) -> (junction 58)
      (junction 58) -> Defrst [order 1] : [DfrstReq]
      (junction 58) -> DefrstOFF [order 2]
      DefrstOFF -> Defrst : [DfrstReq]
      Defrst -> DefrstOFF : [!DfrstReq]
    (default) -> ACOFF
    ACOFF -> ACON : [CabinMode>2&&....
        | (CabinMode!=10||....
        | ACSubMode!=1)]
    ACON -> ACOFF : [CabinMode<=2||....
        | (CabinMode==10&&....
        | ACSubMode==1)]
  state VBase [parallel]
    settings: executionOrder=1
    state Cooling
      en:Vbase=VbaseC;
      du:Vbase=VbaseC;
    state Dehumidity
      en:Vbase=VbaseD;
      du:Vbase=VbaseD;
    state Heating
      en:Vbase=VbaseH;
      du:Vbase=VbaseH;
    state Vmanual
      en:Vbase=Vmanual;
      du:Vbase=Vmanual;
    (default) -> (junction 250)
    (junction 254) -> Cooling [order 1] : [CabinMode==3||....
        | (CabinMode==6&&ACSubMode==2)]
    VBase -> (junction 250) : [hasChanged(CabinMode)||....
        | hasChanged(ACAuto)]
    (junction 250) -> (junction 254) [order 1] : [ACAuto]
    (junction 250) -> Vmanual [order 2]
    (junction 254) -> (junction 258) [order 2]
    (junction 258) -> Dehumidity [order 1] : [CabinMode>3&&CabinMode<8]
    (junction 258) -> (junction 263) [order 2]
    (junction 263) -> Heating [order 1] : [CabinMode>=8]
    (junction 263) -> Vmanual [order 2]
  data: ACAuto input; ACSubMode input; CabinMode input; DfrstReq input; VbaseC input; VbaseD input; VbaseH input; Vmanual input; Vbase local double; Voffset output; PwrSta input; KTHC_VBlowerdfog_K input; KTHC_VBlowerMin_K input; KTHC_VBlowerMid_K input; KTHC_VBlowerDcCh_K input; KTHC_VBlowerSetLow_K input

== stateflow chart thc/THC/ThermalControl/THCM_Conctrl/CompCtrl/Enabled Subsystem/Chart ==
  state LV1
    en:DTymin=KTHC_DTymin1_K;
  state LV2
    en:DTymin=KTHC_DTymin2_K;
  state LV3
    en:DTymin=KTHC_DTymin3_K;
  state LV4
    en:DTymin=KTHC_DTymin4_K;
  state LV5
    en:DTymin=KTHC_DTymin5_K;
  (default) -> (junction 8)
  (junction 8) -> LV1 [order 1] : [Tamb<KTHC_T1Maxamb_C]
  (junction 8) -> (junction 9) [order 2]
  LV1 -> LV2 : [Tamb>KTHC_T1Maxamb_C]
  LV2 -> LV1 [order 2] : [Tamb<KTHC_T2Minamb_C]
  (junction 9) -> LV2 [order 1] : [Tamb<KTHC_T2Maxamb_C]
  (junction 9) -> (junction 10) [order 2]
  LV2 -> LV3 [order 1] : [Tamb>KTHC_T2Maxamb_C]
  LV3 -> LV2 [order 2] : [Tamb<KTHC_T3Minamb_C]
  (junction 10) -> LV3 [order 1] : [Tamb<KTHC_T3Maxamb_C]
  (junction 10) -> (junction 11) [order 2]
  LV3 -> LV4 [order 1] : [Tamb>KTHC_T3Maxamb_C]
  LV4 -> LV3 [order 2] : [Tamb<KTHC_T4Minamb_C]
  (junction 11) -> LV4 [order 1] : [Tamb<KTHC_T4Maxamb_C]
  (junction 11) -> (junction 12) [order 2]
  LV4 -> LV5 [order 1] : [Tamb>KTHC_T4Maxamb_C]
  LV5 -> LV4 : [Tamb<KTHC_T5Minamb_C]
  (junction 12) -> LV5
  data: Tamb input; KTHC_DTymin1_K input; KTHC_DTymin2_K input; KTHC_DTymin3_K input; KTHC_DTymin4_K input; KTHC_DTymin5_K input; KTHC_T1Maxamb_C input; KTHC_T2Maxamb_C input; KTHC_T3Maxamb_C input; KTHC_T4Maxamb_C input; KTHC_T2Minamb_C input; KTHC_T3Minamb_C input; KTHC_T4Minamb_C input; KTHC_T5Minamb_C input; DTymin output double

== stateflow chart thc/THC/ThermalControl/THCM_Conctrl/APTC/Chart ==
  state APTCPro_FrLe [parallel]
    settings: executionOrder=1
    state Derating
      state State2
        (default) -> (junction 23)
        APTCPro_FrLe.Derating.State2 -> (junction 23) [order 1]
        (junction 23) -> (junction 26) [order 1] : [FD_FrLeAPTCHeatPwr_Cmd>KTHC_DAPTCQ1_W]{FD_FrLeAPTCHeatPwr_Cmd=FD_FrLeAPTCHeatPwr_Cmd-KTHC_DAPTCQ1_W;}
        (junction 23) -> (junction 28) [order 2] : {FD_FrLeAPTCHeatPwr_Cmd=0;}
      state State3
        (default) -> (junction 31)
        APTCPro_FrLe.Derating.State3 -> (junction 31) [order 1]
        (junction 31) -> (junction 32) [order 1] : [FD_FrLeAPTCHeatPwr_Cmd>KTHC_DAPTCQ2_W]{FD_FrLeAPTCHeatPwr_Cmd=FD_FrLeAPTCHeatPwr_Cmd-KTHC_DAPTCQ2_W;}
        (junction 31) -> (junction 33) [order 2] : {FD_FrLeAPTCHeatPwr_Cmd=0;}
      state State4
        (default) -> (junction 39)
        APTCPro_FrLe.Derating.State4 -> (junction 39) [order 1]
        (junction 39) -> (junction 40) [order 1] : [FD_FrLeAPTCHeatPwr_Cmd>KTHC_DAPTCQ3_W]{FD_FrLeAPTCHeatPwr_Cmd=FD_FrLeAPTCHeatPwr_Cmd-KTHC_DAPTCQ3_W;}
        (junction 39) -> (junction 41) [order 2] : {FD_FrLeAPTCHeatPwr_Cmd=0;}
      state State5
      (default) -> APTCPro_FrLe.Derating.State2
      APTCPro_FrLe.Derating.State3 -> APTCPro_FrLe.Derating.State2 [order 1] : [Tventmax_FrLe>KTHC_TventL1_C]
      APTCPro_FrLe.Derating.State2 -> APTCPro_FrLe.Derating.State3 [order 1] : [Tventmax_FrLe<KTHC_TventL2_C]
      APTCPro_FrLe.Derating.State4 -> APTCPro_FrLe.Derating.State3 [order 1] : [Tventmax_FrLe>KTHC_TventL2_C]
      APTCPro_FrLe.Derating.State3 -> APTCPro_FrLe.Derating.State4 [order 2] : [Tventmax_FrLe<KTHC_TventL3_C]
      APTCPro_FrLe.Derating.State5 -> APTCPro_FrLe.Derating.State4 : [Tventmax_FrLe>KTHC_TventL3_C]
      APTCPro_FrLe.Derating.State4 -> APTCPro_FrLe.Derating.State5 [order 2] : [Tventmax_FrLe<KTHC_TventL4_C]
    state PICtrl
      en:FD_FrLeAPTCHeatPwr_Cmd=FD_FrLeAPTC_Cmd;
      du:FD_FrLeAPTCHeatPwr_Cmd=FD_FrLeAPTC_Cmd;
      state Normal
        en:CtrlReset=0;
      state ResetController
        en:CtrlReset=1;
      (default) -> APTCPro_FrLe.PICtrl.Normal
      APTCPro_FrLe.PICtrl.ResetController -> APTCPro_FrLe.PICtrl.Normal
    (default) -> APTCPro_FrLe.PICtrl
    APTCPro_FrLe.PICtrl -> APTCPro_FrLe.Derating : [Tventmax_FrLe>KTHC_TventL1_C]
    APTCPro_FrLe.Derating -> APTCPro_FrLe.PICtrl [order 2] : [FD_FrLeAPTCHeatPwr_Cmd>FD_FrLeAPTC_Cmd]
    APTCPro_FrLe.Derating -> APTCPro_FrLe.PICtrl.ResetController [order 1] : [Tventmax_FrLe<KTHC_TventL5_C]
  state APTCPro_FrRi [parallel]
    settings: executionOrder=2
    state Derating
      state State2
        (default) -> (junction 87)
        APTCPro_FrRi.Derating.State2 -> (junction 87) [order 1]
        (junction 87) -> (junction 88) [order 1] : [FD_FrRiAPTCHeatPwr_Cmd>KTHC_DAPTCQ1_W]{FD_FrRiAPTCHeatPwr_Cmd=FD_FrRiAPTCHeatPwr_Cmd-KTHC_DAPTCQ1_W;}
        (junction 87) -> (junction 89) [order 2] : {FD_FrRiAPTCHeatPwr_Cmd=0;}
      state State3
        (default) -> (junction 58)
        APTCPro_FrRi.Derating.State3 -> (junction 58) [order 1]
        (junction 58) -> (junction 59) [order 1] : [FD_FrRiAPTCHeatPwr_Cmd>KTHC_DAPTCQ2_W]{FD_FrRiAPTCHeatPwr_Cmd=FD_FrRiAPTCHeatPwr_Cmd-KTHC_DAPTCQ2_W;}
        (junction 58) -> (junction 60) [order 2] : {FD_FrRiAPTCHeatPwr_Cmd=0;}
      state State4
        (default) -> (junction 78)
        APTCPro_FrRi.Derating.State4 -> (junction 78) [order 1]
        (junction 78) -> (junction 79) [order 1] : [FD_FrRiAPTCHeatPwr_Cmd>KTHC_DAPTCQ3_W]{FD_FrRiAPTCHeatPwr_Cmd=FD_FrRiAPTCHeatPwr_Cmd-KTHC_DAPTCQ3_W;}
        (junction 78) -> (junction 80) [order 2] : {FD_FrRiAPTCHeatPwr_Cmd=0;}
      state State5
      (default) -> APTCPro_FrRi.Derating.State2
      APTCPro_FrRi.Derating.State3 -> APTCPro_FrRi.Derating.State2 [order 1] : [Tventmax_FrRi>KTHC_TventL1_C]
      APTCPro_FrRi.Derating.State2 -> APTCPro_FrRi.Derating.State3 [order 1] : [Tventmax_FrRi<KTHC_TventL2_C]
      APTCPro_FrRi.Derating.State4 -> APTCPro_FrRi.Derating.State3 [order 1] : [Tventmax_FrRi>KTHC_TventL2_C]
      APTCPro_FrRi.Derating.State3 -> APTCPro_FrRi.Derating.State4 [order 2] : [Tventmax_FrRi<KTHC_TventL3_C]
      APTCPro_FrRi.Derating.State5 -> APTCPro_FrRi.Derating.State4 : [Tventmax_FrRi>KTHC_TventL3_C]
      APTCPro_FrRi.Derating.State4 -> APTCPro_FrRi.Derating.State5 [order 2] : [Tventmax_FrRi<KTHC_TventL4_C]
    state PICtrl
      en:FD_FrRiAPTCHeatPwr_Cmd=FD_FrRiAPTC_Cmd;
      du:FD_FrRiAPTCHeatPwr_Cmd=FD_FrRiAPTC_Cmd;
      state Normal
        en:CtrlReset=0;
      state ResetController
        en:CtrlReset=1;
      (default) -> APTCPro_FrRi.PICtrl.Normal
      APTCPro_FrRi.PICtrl.ResetController -> APTCPro_FrRi.PICtrl.Normal
    (default) -> APTCPro_FrRi.PICtrl
    APTCPro_FrRi.PICtrl -> APTCPro_FrRi.Derating : [Tventmax_FrRi>KTHC_TventL1_C]
    APTCPro_FrRi.Derating -> APTCPro_FrRi.PICtrl [order 2] : [FD_FrRiAPTCHeatPwr_Cmd>FD_FrRiAPTC_Cmd]
    APTCPro_FrRi.Derating -> APTCPro_FrRi.PICtrl.ResetController [order 1] : [Tventmax_FrRi<KTHC_TventL5_C]
  state APTCPro_Rr [parallel]
    settings: executionOrder=3
    state Derating
      state State2
        (default) -> (junction 125)
        APTCPro_Rr.Derating.State2 -> (junction 125) [order 1]
        (junction 125) -> (junction 126) [order 1] : [FD_RrAPTCHeatPwr_Cmd>KTHC_DAPTCQ1_W]{FD_RrAPTCHeatPwr_Cmd=FD_RrAPTCHeatPwr_Cmd-KTHC_DAPTCQ1_W;}
        (junction 125) -> (junction 127) [order 2] : {FD_RrAPTCHeatPwr_Cmd=0;}
      state State3
        (default) -> (junction 96)
        APTCPro_Rr.Derating.State3 -> (junction 96) [order 1]
        (junction 96) -> (junction 97) [order 1] : [FD_RrAPTCHeatPwr_Cmd>KTHC_DAPTCQ2_W]{FD_RrAPTCHeatPwr_Cmd=FD_RrAPTCHeatPwr_Cmd-KTHC_DAPTCQ2_W;}
        (junction 96) -> (junction 98) [order 2] : {FD_RrAPTCHeatPwr_Cmd=0;}
      state State4
        (default) -> (junction 116)
        APTCPro_Rr.Derating.State4 -> (junction 116) [order 1]
        (junction 116) -> (junction 117) [order 1] : [FD_RrAPTCHeatPwr_Cmd>KTHC_DAPTCQ3_W]{FD_RrAPTCHeatPwr_Cmd=FD_RrAPTCHeatPwr_Cmd-KTHC_DAPTCQ3_W;}
        (junction 116) -> (junction 118) [order 2] : {FD_RrAPTCHeatPwr_Cmd=0;}
      state State5
      (default) -> APTCPro_Rr.Derating.State2
      APTCPro_Rr.Derating.State3 -> APTCPro_Rr.Derating.State2 [order 1] : [Tventmax_Rr>KTHC_TventL1_C]
      APTCPro_Rr.Derating.State2 -> APTCPro_Rr.Derating.State3 [order 1] : [Tventmax_Rr<KTHC_TventL2_C]
      APTCPro_Rr.Derating.State4 -> APTCPro_Rr.Derating.State3 [order 1] : [Tventmax_Rr>KTHC_TventL2_C]
      APTCPro_Rr.Derating.State3 -> APTCPro_Rr.Derating.State4 [order 2] : [Tventmax_Rr<KTHC_TventL3_C]
      APTCPro_Rr.Derating.State5 -> APTCPro_Rr.Derating.State4 : [Tventmax_Rr>KTHC_TventL3_C]
      APTCPro_Rr.Derating.State4 -> APTCPro_Rr.Derating.State5 [order 2] : [Tventmax_Rr<KTHC_TventL4_C]
    state PICtrl
      en:FD_RrAPTCHeatPwr_Cmd=FD_RrAPTC_Cmd;
      du:FD_RrAPTCHeatPwr_Cmd=FD_RrAPTC_Cmd;
      state Normal
        en:CtrlReset=0;
      state ResetController
        en:CtrlReset=1;
      (default) -> APTCPro_Rr.PICtrl.Normal
      APTCPro_Rr.PICtrl.ResetController -> APTCPro_Rr.PICtrl.Normal
    (default) -> APTCPro_Rr.PICtrl
    APTCPro_Rr.PICtrl -> APTCPro_Rr.Derating : [Tventmax_Rr>KTHC_TventL1_C]
    APTCPro_Rr.Derating -> APTCPro_Rr.PICtrl [order 2] : [FD_RrAPTCHeatPwr_Cmd>FD_RrAPTC_Cmd]
    APTCPro_Rr.Derating -> APTCPro_Rr.PICtrl.ResetController [order 1] : [Tventmax_Rr<KTHC_TventL5_C]
  data: FD_FrLeAPTC_Cmd input; FD_FrRiAPTC_Cmd input; FD_RrAPTC_Cmd input; Tventmax_FrLe input; Tventmax_FrRi input; Tventmax_Rr input; KTHC_TventL1_C input; KTHC_TventL2_C input; KTHC_TventL3_C input; KTHC_TventL4_C input; KTHC_TventL5_C input; KTHC_DAPTCQ1_W input; KTHC_DAPTCQ2_W input; KTHC_DAPTCQ3_W input; FD_FrLeAPTCHeatPwr_Cmd output double; FD_FrRiAPTCHeatPwr_Cmd output double; FD_RrAPTCHeatPwr_Cmd output double; CtrlReset output boolean
